simulink model "four_machine"  (R2020a)
settings: Solver=ode15s  StartTime=0.0  StopTime=20  MaxStep=1/60  RelTol=1e-3  EnableMultiTasking=on
values from neighbouring files (symbols this model uses):
  case_n = i-1    [main_simulations.m]
  d11_step = load_step_size    (= 350)    [main_simulations.m]
  d5_step = 0    [main_simulations.m]
  H = [6.5 6.5 6.175 6.175]*.75    [main_simulations.m]
  kpss = 0.2    [main_simulations.m]
  Tdelay = 0.2    [main_simulations.m]
undefined symbols (not defined in the file or in its folder): D1, d_rad, Delta, K
libraries: powerlib x49, sps_avr x4, powerlib_meascontrol x4, simulink x2, dspsigops x2
(part 2 of 2)

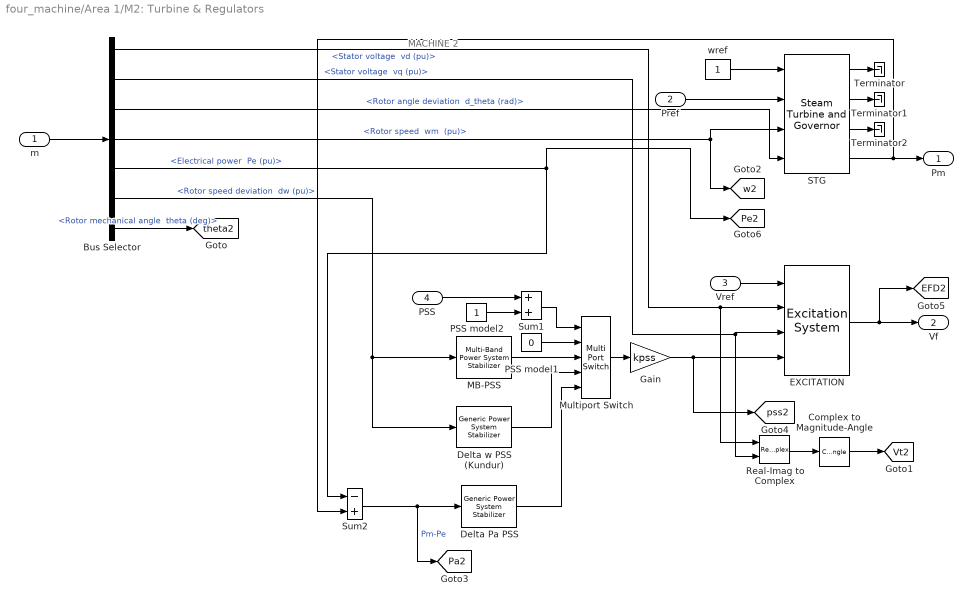
== system four_machine/Area 1/M2: Turbine & Regulators ==
  note: MACHINE 2
  m : Inport
  Pref : Inport  Port=2
  Vref : Inport  Port=3
  PSS : Inport  Port=4
  Bus Selector : BusSelector  OutputSignals="dq0 components.Stator voltage  vd (pu),dq0 components.Stator voltage  vq (pu),Mechanical.Rotor angle deviation  d_theta (rad),Mechanical.Rotor speed  wm  (pu),Mechanical.Electrical power  Pe (pu),Mechanical.Rotor speed deviation  dw (pu),Mechanical.Rotor mechanical angle  theta (deg)"
  Complex to Magnitude-Angle : ComplexToMagnitudeAngle  Output=Magnitude
  "Delta Pa PSS " : powerlib/Machines/Generic Power System Stabilizer  Tsensor=15e-3  K=2.5*1.25  Twashout=1  Tleadlag1=[60e-3 1]  Tleadlag2=[0 0]  VSlimits=[-0.15 0.15]  Vinit=0  Plot_On=off  MagdB_On=on  FreqRange=logspace(-2,2,500)
      settings: SourceProductBaseCode=PS
  "Delta w PSS (Kundur) " : powerlib/Machines/Generic Power System Stabilizer  Tsensor=15e-3  K=30  Twashout=10  Tleadlag1=[50e-3 20e-3]  Tleadlag2=[3 5.4]  VSlimits=[-0.15 0.15]  Vinit=0  Plot_On=off  MagdB_On=on  FreqRange=logspace(-2,2,500)
      settings: SourceProductBaseCode=PS
  EXCITATION : sps_avr/Excitation System  tr=20e-3  reg=[ 200, 0.001 ]  exc=[ 1, 0 ]  tgr=[ 0, 0 ]  damp=[ 0, 0 ]  sat=[ 0, 0 ]  lim=[ 0 , 12.3, 0 ]  v0=[1 2.1188]
      settings: SourceProductBaseCode=PS
  Gain : Gain  Gain=kpss
  "MB-PSS " : powerlib/Machines/Multi-Band Power System Stabilizer  OperationMode=Simplified settings  Kg=1.0  GL=[0.2 30]  GI=[1.25 40]  GH=[12.0 160]  GLd=[66 66 9.4]  TcLF=[1.667 2 0 0 0 0 2 2.4 0 0 0 0 1 1]  GId=[66 66 47.6]  TcIF=[1 1 0.25 0.3 0 0 1 1 0.3 0.36 0 0 0 0]  GHd=[66 66 233]  TcHF="[0.01 0.012 0 0 0 0  0.012 0.0144 0 0 0 0 1 1]"  LIM=[.075 .15 .15 .15]  Plot_On=off  MagdB_On=off  FreqRange=logspace(-2,2,500)
      settings: SourceProductBaseCode=PS
  Multiport Switch : MultiPortSwitch  Inputs=4  InputSameDT=on
  PSS model1 : Constant  Value=0
  PSS model2 : Constant
  Real-Imag to Complex : RealImagToComplex
  STG : powerlib/Machines/Steam Turbine and Governor  gentype=Tandem-compound (single mass)  reg1="[ 1  0.05    0 ]"  reg2="[ 0.001  0.15 ]"  reg3="[ -0.1  0.1  0  4.496 ]"  N=3600  turb1="[ 0  10   3.3   0.5   ]"  turb2="[   0   0.36    0.36   0.28   ]"  HA="[ 0.046  1.430  1.465   0.192 ]"  KA="[ 90.44  53.88  64.59   62.94  ]"  DA="[ 0.0115  0.3575  0.3663   0.0137  ]"  ini1=0.86358  ini2=[0.779243,-42.8075]
      settings: SourceProductBaseCode=PS
  Sum1 : Sum  InputSameDT=on  SaturateOnIntegerOverflow=on  OutDataTypeStr=Inherit: Same as first input
  Sum2 : Sum  Inputs=-+  InputSameDT=on  SaturateOnIntegerOverflow=on  OutDataTypeStr=Inherit: Same as first input
  Terminator : Terminator
  Terminator1 : Terminator
  Terminator2 : Terminator
  wref : Constant
  Pm : Outport  InitialOutput=0  VectorParamsAs1DForOutWhenUnconnected=off
  Vf : Outport  Port=2  InitialOutput=0  VectorParamsAs1DForOutWhenUnconnected=off
  tag scope: EFD2=global, Pa2=global, Pe2=global, Vt2=global, pss2=global, theta2=global, w2=global
  wires:
  Sum2/1 -> [Pa2], "Delta Pa PSS "/1  "Pm-Pe"
  Bus Selector/6 -> "MB-PSS "/1, "Delta w PSS (Kundur) "/1  "<Rotor speed deviation  dw (pu)>"
  Bus Selector/5 -> [Pe2], Sum2/1  "<Electrical power  Pe (pu)>"
  Bus Selector/4 -> STG/3, [w2]  "<Rotor speed  wm  (pu)>"
  PSS/1 -> Sum1/1
  Sum1/1 -> Multiport Switch/1
  PSS model2/1 -> Sum1/2
  "Delta Pa PSS "/1 -> Multiport Switch/5
  "Delta w PSS (Kundur) "/1 -> Multiport Switch/4
  "MB-PSS "/1 -> Multiport Switch/3
  PSS model1/1 -> Multiport Switch/2
  Multiport Switch/1 -> Gain/1
  Bus Selector/7 -> [theta2]  "<Rotor mechanical angle  theta (deg)>"
  Complex to Magnitude-Angle/1 -> [Vt2]
  EXCITATION/1 -> [EFD2], Vf/1
  Real-Imag to Complex/1 -> Complex to Magnitude-Angle/1
  Vref/1 -> EXCITATION/1
  Pref/1 -> STG/2
  wref/1 -> STG/1
  Bus Selector/2 -> Real-Imag to Complex/2, EXCITATION/3  "<Stator voltage  vq (pu)>"
  Bus Selector/1 -> Real-Imag to Complex/1, EXCITATION/2  "<Stator voltage  vd (pu)>"
  STG/1 -> Terminator/1
  STG/2 -> Terminator1/1
  STG/3 -> Terminator2/1
  STG/4 -> Pm/1, Sum2/2
  Bus Selector/3 -> STG/4  "<Rotor angle deviation  d_theta (rad)>"
  m/1 -> Bus Selector/1
  Gain/1 -> [pss2], EXCITATION/4

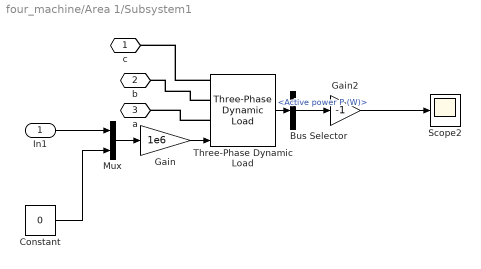
== system four_machine/Area 1/Subsystem1 ==
  In1 : Inport
  Bus Selector : BusSelector  OutputSignals=Active power P (W)
  Constant : Constant  Value=0
  Gain : Gain  Gain=1e6
  Gain2 : Gain  Gain=-1
  Mux : Mux  Inputs=2
  Scope2 : Scope
  Three-Phase Dynamic Load : powerlib/Elements/Three-Phase Dynamic Load  NominalVoltage=[ 230e3 60 ]  ActiveReactivePowers=[1e-06 1e-06]  PositiveSequence=[0.985471 32.8037]  ExternalControl=on  NpNq=[1.3 2]  TimeConstants="[0  0  0  0]"  MinimumVoltage=0.7  Tfilter=1e-4  LoadFlowParameters=[4,0,0,0,0]
      settings: SourceProductBaseCode=PS
  c : PMIOPort  Side=Left
  b : PMIOPort  Port=2  Side=Left
  a : PMIOPort  Port=3  Side=Left
  wires:
  Bus Selector/1 -> Gain2/1  "<Active power P (W)>"
  Three-Phase Dynamic Load/1 -> Bus Selector/1
  Mux/1 -> Gain/1
  Constant/1 -> Mux/2
  Gain/1 -> Three-Phase Dynamic Load/1
  In1/1 -> Mux/1
  Gain2/1 -> Scope2/1
  connections:
  Three-Phase Dynamic Load/LConn2 -- b/RConn1
  Three-Phase Dynamic Load/LConn3 -- c/RConn1
  Three-Phase Dynamic Load/LConn1 -- a/RConn1

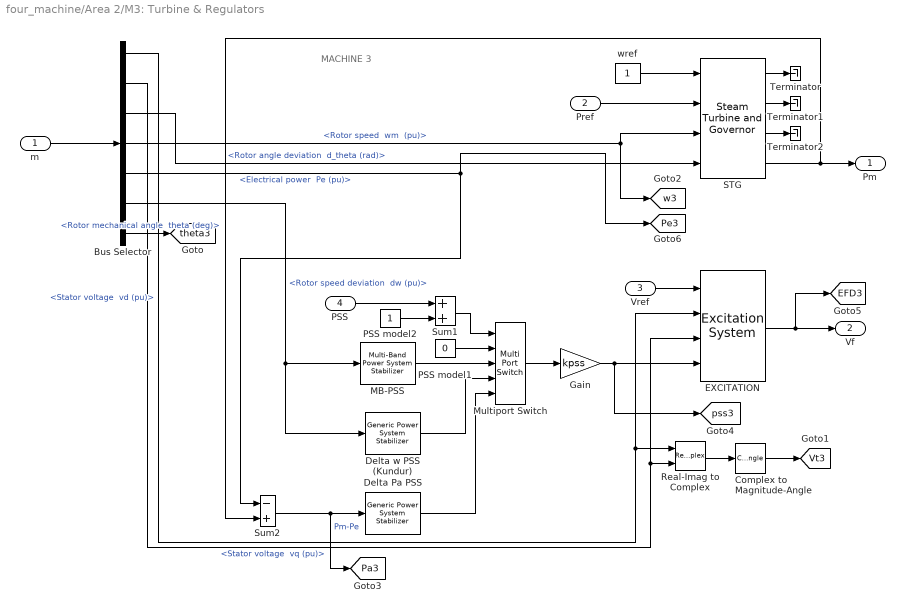
== system four_machine/Area 2/M3: Turbine & Regulators ==
  note: MACHINE 3
  m : Inport
  Pref : Inport  Port=2
  Vref : Inport  Port=3
  PSS : Inport  Port=4
  Bus Selector : BusSelector  OutputSignals="dq0 components.Stator voltage  vd (pu),dq0 components.Stator voltage  vq (pu),Mechanical.Rotor angle deviation  d_theta (rad),Mechanical.Rotor speed  wm  (pu),Mechanical.Electrical power  Pe (pu),Mechanical.Rotor speed deviation  dw (pu),Mechanical.Rotor mechanical angle  theta (deg)"
  Complex to Magnitude-Angle : ComplexToMagnitudeAngle  Output=Magnitude
  "Delta Pa PSS " : powerlib/Machines/Generic Power System Stabilizer  Tsensor=15e-3  K=2.5*1.25  Twashout=1  Tleadlag1=[60e-3 1]  Tleadlag2=[0 0]  VSlimits=[-0.15 0.15]  Vinit=0  Plot_On=off  MagdB_On=on  FreqRange=logspace(-2,2,500)
      settings: SourceProductBaseCode=PS
  "Delta w PSS (Kundur) " : powerlib/Machines/Generic Power System Stabilizer  Tsensor=15e-3  K=30  Twashout=10  Tleadlag1=[50e-3 20e-3]  Tleadlag2=[3 5.4]  VSlimits=[-0.15 0.15]  Vinit=0  Plot_On=off  MagdB_On=on  FreqRange=logspace(-2,2,500)
      settings: SourceProductBaseCode=PS
  EXCITATION : sps_avr/Excitation System  tr=20e-3  reg=[ 200, 0.001 ]  exc=[ 1, 0 ]  tgr=[ 0, 0 ]  damp=[ 0, 0 ]  sat=[ 0, 0 ]  lim=[ 0 , 12.3, 0 ]  v0=[1 1.8982]
      settings: SourceProductBaseCode=PS
  Gain : Gain  Gain=kpss
  "MB-PSS " : powerlib/Machines/Multi-Band Power System Stabilizer  OperationMode=Simplified settings  Kg=1.0  GL=[0.2 30]  GI=[1.25 40]  GH=[12.0 160]  GLd=[66 66 9.4]  TcLF=[1.667 2 0 0 0 0 2 2.4 0 0 0 0 1 1]  GId=[66 66 47.6]  TcIF=[1 1 0.25 0.3 0 0 1 1 0.3 0.36 0 0 0 0]  GHd=[66 66 233]  TcHF="[0.01 0.012 0 0 0 0  0.012 0.0144 0 0 0 0 1 1]"  LIM=[.075 .15 .15 .15]  Plot_On=off  MagdB_On=off  FreqRange=logspace(-2,2,500)
      settings: SourceProductBaseCode=PS
  Multiport Switch : MultiPortSwitch  Inputs=4  InputSameDT=on
  PSS model1 : Constant  Value=0
  PSS model2 : Constant
  Real-Imag to Complex : RealImagToComplex
  STG : powerlib/Machines/Steam Turbine and Governor  gentype=Tandem-compound (single mass)  reg1="[ 1  0.05    0 ]"  reg2="[ 0.001  0.15 ]"  reg3="[ -0.1  0.1  0  4.496 ]"  N=3600  turb1="[ 0  10   3.3   0.5   ]"  turb2="[   0   0.36    0.36   0.28   ]"  HA="[ 0.046  1.430  1.465   0.192 ]"  KA="[ 90.44  53.88  64.59   62.94  ]"  DA="[ 0.0115  0.3575  0.3663   0.0137  ]"  ini1=0.80053  ini2=[0.800505,-56.3243]
      settings: SourceProductBaseCode=PS
  Sum1 : Sum  InputSameDT=on  SaturateOnIntegerOverflow=on  OutDataTypeStr=Inherit: Same as first input
  Sum2 : Sum  Inputs=-+  InputSameDT=on  SaturateOnIntegerOverflow=on  OutDataTypeStr=Inherit: Same as first input
  Terminator : Terminator
  Terminator1 : Terminator
  Terminator2 : Terminator
  wref : Constant
  Pm : Outport  InitialOutput=0  VectorParamsAs1DForOutWhenUnconnected=off
  Vf : Outport  Port=2  InitialOutput=0  VectorParamsAs1DForOutWhenUnconnected=off
  tag scope: EFD3=global, Pa3=global, Pe3=global, Vt3=global, pss3=global, theta3=global, w3=global
  wires:
  Sum2/1 -> [Pa3], "Delta Pa PSS "/1  "Pm-Pe"
  Bus Selector/6 -> "MB-PSS "/1, "Delta w PSS (Kundur) "/1  "<Rotor speed deviation  dw (pu)>"
  Bus Selector/5 -> [Pe3], Sum2/1  "<Electrical power  Pe (pu)>"
  Bus Selector/4 -> STG/3, [w3]  "<Rotor speed  wm  (pu)>"
  PSS/1 -> Sum1/1
  Sum1/1 -> Multiport Switch/1
  PSS model2/1 -> Sum1/2
  "Delta Pa PSS "/1 -> Multiport Switch/5
  "Delta w PSS (Kundur) "/1 -> Multiport Switch/4
  "MB-PSS "/1 -> Multiport Switch/3
  PSS model1/1 -> Multiport Switch/2
  Multiport Switch/1 -> Gain/1
  Bus Selector/7 -> [theta3]  "<Rotor mechanical angle  theta (deg)>"
  Complex to Magnitude-Angle/1 -> [Vt3]
  EXCITATION/1 -> [EFD3], Vf/1
  Real-Imag to Complex/1 -> Complex to Magnitude-Angle/1
  Vref/1 -> EXCITATION/1
  Pref/1 -> STG/2
  wref/1 -> STG/1
  Bus Selector/2 -> EXCITATION/3, Real-Imag to Complex/2  "<Stator voltage  vq (pu)>"
  Bus Selector/1 -> EXCITATION/2, Real-Imag to Complex/1  "<Stator voltage  vd (pu)>"
  Bus Selector/3 -> STG/4  "<Rotor angle deviation  d_theta (rad)>"
  STG/1 -> Terminator/1
  STG/2 -> Terminator1/1
  STG/3 -> Terminator2/1
  STG/4 -> Pm/1, Sum2/2
  m/1 -> Bus Selector/1
  Gain/1 -> [pss3], EXCITATION/4

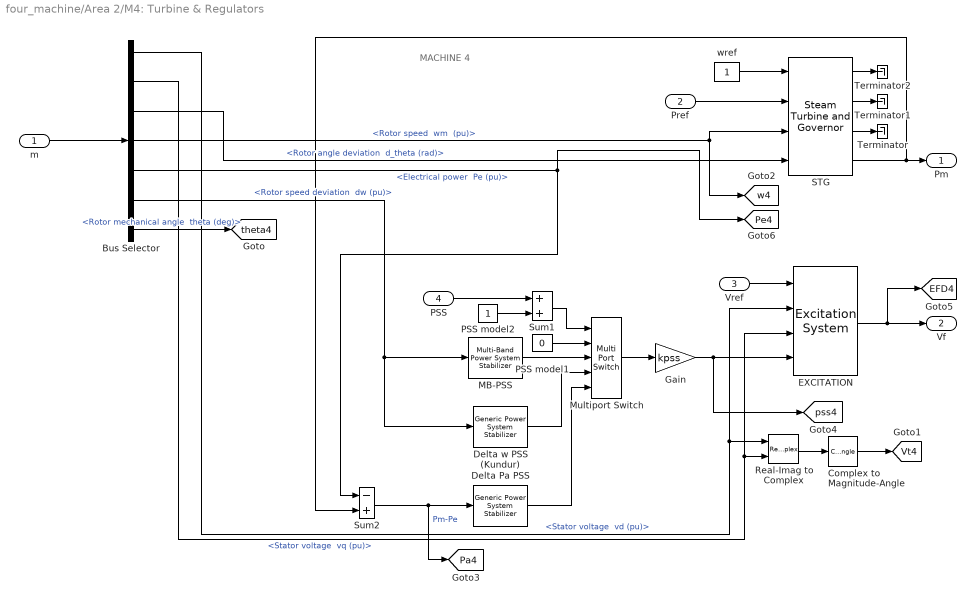
== system four_machine/Area 2/M4: Turbine & Regulators ==
  note: MACHINE 4
  m : Inport
  Pref : Inport  Port=2
  Vref : Inport  Port=3
  PSS : Inport  Port=4
  Bus Selector : BusSelector  OutputSignals="dq0 components.Stator voltage  vd (pu),dq0 components.Stator voltage  vq (pu),Mechanical.Rotor angle deviation  d_theta (rad),Mechanical.Rotor speed  wm  (pu),Mechanical.Electrical power  Pe (pu),Mechanical.Rotor speed deviation  dw (pu),Mechanical.Rotor mechanical angle  theta (deg)"
  Complex to Magnitude-Angle : ComplexToMagnitudeAngle  Output=Magnitude
  "Delta Pa PSS " : powerlib/Machines/Generic Power System Stabilizer  Tsensor=15e-3  K=2.5*1.25  Twashout=1  Tleadlag1=[60e-3 1]  Tleadlag2=[0 0]  VSlimits=[-0.15 0.15]  Vinit=0  Plot_On=off  MagdB_On=on  FreqRange=logspace(-2,2,500)
      settings: SourceProductBaseCode=PS
  "Delta w PSS (Kundur) " : powerlib/Machines/Generic Power System Stabilizer  Tsensor=15e-3  K=30  Twashout=10  Tleadlag1=[50e-3 20e-3]  Tleadlag2=[3 5.4]  VSlimits=[-0.15 0.15]  Vinit=0  Plot_On=off  MagdB_On=on  FreqRange=logspace(-2,2,500)
      settings: SourceProductBaseCode=PS
  EXCITATION : sps_avr/Excitation System  tr=20e-3  reg=[ 200, 0.001 ]  exc=[ 1, 0 ]  tgr=[ 0, 0 ]  damp=[ 0, 0 ]  sat=[ 0, 0 ]  lim=[ 0 , 12.3, 0 ]  v0=[1 1.9423]
      settings: SourceProductBaseCode=PS
  Gain : Gain  Gain=kpss
  "MB-PSS " : powerlib/Machines/Multi-Band Power System Stabilizer  OperationMode=Simplified settings  Kg=1.0  GL=[0.2 30]  GI=[1.25 40]  GH=[12.0 160]  GLd=[66 66 9.4]  TcLF=[1.667 2 0 0 0 0 2 2.4 0 0 0 0 1 1]  GId=[66 66 47.6]  TcIF=[1 1 0.25 0.3 0 0 1 1 0.3 0.36 0 0 0 0]  GHd=[66 66 233]  TcHF="[0.01 0.012 0 0 0 0  0.012 0.0144 0 0 0 0 1 1]"  LIM=[.075 .15 .15 .15]  Plot_On=off  MagdB_On=off  FreqRange=logspace(-2,2,500)
      settings: SourceProductBaseCode=PS
  Multiport Switch : MultiPortSwitch  Inputs=4  InputSameDT=on
  PSS model1 : Constant  Value=0
  PSS model2 : Constant
  Real-Imag to Complex : RealImagToComplex
  STG : powerlib/Machines/Steam Turbine and Governor  gentype=Tandem-compound (single mass)  reg1="[ 1  0.05    0 ]"  reg2="[ 0.001  0.15 ]"  reg3="[ -0.1  0.1  0  4.496 ]"  N=3600  turb1="[ 0  10   3.3   0.5   ]"  turb2="[   0   0.36    0.36   0.28   ]"  HA="[ 0.046  1.430  1.465   0.192 ]"  KA="[ 90.44  53.88  64.59   62.94  ]"  DA="[ 0.0115  0.3575  0.3663   0.0137  ]"  ini1=0.77938  ini2=[0.779311,-67.7513]
      settings: SourceProductBaseCode=PS
  Sum1 : Sum  InputSameDT=on  SaturateOnIntegerOverflow=on  OutDataTypeStr=Inherit: Same as first input
  Sum2 : Sum  Inputs=-+  InputSameDT=on  SaturateOnIntegerOverflow=on  OutDataTypeStr=Inherit: Same as first input
  Terminator : Terminator
  Terminator1 : Terminator
  Terminator2 : Terminator
  wref : Constant
  Pm : Outport  InitialOutput=0  VectorParamsAs1DForOutWhenUnconnected=off
  Vf : Outport  Port=2  InitialOutput=0  VectorParamsAs1DForOutWhenUnconnected=off
  tag scope: EFD4=global, Pa4=global, Pe4=global, Vt4=global, pss4=global, theta4=global, w4=global
  wires:
  Bus Selector/1 -> EXCITATION/2, Real-Imag to Complex/1  "<Stator voltage  vd (pu)>"
  Bus Selector/2 -> EXCITATION/3, Real-Imag to Complex/2  "<Stator voltage  vq (pu)>"
  STG/4 -> Pm/1, Sum2/2
  wref/1 -> STG/1
  Pref/1 -> STG/2
  Vref/1 -> EXCITATION/1
  STG/3 -> Terminator/1
  Real-Imag to Complex/1 -> Complex to Magnitude-Angle/1
  EXCITATION/1 -> Vf/1, [EFD4]
  Complex to Magnitude-Angle/1 -> [Vt4]
  Bus Selector/7 -> [theta4]  "<Rotor mechanical angle  theta (deg)>"
  Multiport Switch/1 -> Gain/1
  PSS model1/1 -> Multiport Switch/2
  "MB-PSS "/1 -> Multiport Switch/3
  "Delta w PSS (Kundur) "/1 -> Multiport Switch/4
  "Delta Pa PSS "/1 -> Multiport Switch/5
  PSS model2/1 -> Sum1/2
  Sum1/1 -> Multiport Switch/1
  PSS/1 -> Sum1/1
  Bus Selector/4 -> STG/3, [w4]  "<Rotor speed  wm  (pu)>"
  Bus Selector/5 -> [Pe4], Sum2/1  "<Electrical power  Pe (pu)>"
  Bus Selector/6 -> "MB-PSS "/1, "Delta w PSS (Kundur) "/1  "<Rotor speed deviation  dw (pu)>"
  Sum2/1 -> [Pa4], "Delta Pa PSS "/1  "Pm-Pe"
  STG/2 -> Terminator1/1
  STG/1 -> Terminator2/1
  Bus Selector/3 -> STG/4  "<Rotor angle deviation  d_theta (rad)>"
  m/1 -> Bus Selector/1
  Gain/1 -> EXCITATION/4, [pss4]

== system four_machine/Area 2/Subsystem1 ==
  In1 : Inport
  Bus Selector : BusSelector  OutputSignals=Active power P (W)
  Constant : Constant  Value=0
  Gain : Gain  Gain=1e6
  Gain2 : Gain  Gain=-1
  Mux : Mux  Inputs=2
  Scope2 : Scope
  Three-Phase Dynamic Load : powerlib/Elements/Three-Phase Dynamic Load  NominalVoltage=[ 230e3 60 ]  ActiveReactivePowers=[1e-06 1e-06]  PositiveSequence=[0.98771 -4.64632]  ExternalControl=on  NpNq=[1.3 2]  TimeConstants="[0  0  0  0]"  MinimumVoltage=0.7  Tfilter=1e-4  LoadFlowParameters=[4,0,0,0,0]
      settings: SourceProductBaseCode=PS
  c : PMIOPort  Side=Left
  b : PMIOPort  Port=2  Side=Left
  a : PMIOPort  Port=3  Side=Left
  wires:
  Bus Selector/1 -> Gain2/1  "<Active power P (W)>"
  Three-Phase Dynamic Load/1 -> Bus Selector/1
  Mux/1 -> Gain/1
  Constant/1 -> Mux/2
  Gain/1 -> Three-Phase Dynamic Load/1
  In1/1 -> Mux/1
  Gain2/1 -> Scope2/1
  connections:
  Three-Phase Dynamic Load/LConn2 -- b/RConn1
  Three-Phase Dynamic Load/LConn3 -- c/RConn1
  Three-Phase Dynamic Load/LConn1 -- a/RConn1

== system four_machine/Subsystem3/Subsystem ==
  u : Inport
  Enable : EnablePort
  y : Outport  VectorParamsAs1DForOutWhenUnconnected=off
  wires:
  u/1 -> y/1

== system four_machine/Subsystem4/Subsystem ==
  u : Inport
  Enable : EnablePort
  y : Outport  VectorParamsAs1DForOutWhenUnconnected=off
  wires:
  u/1 -> y/1

== system four_machine/Subsystem5/Subsystem ==
  u : Inport
  Enable : EnablePort
  y : Outport  VectorParamsAs1DForOutWhenUnconnected=off
  wires:
  u/1 -> y/1

== system four_machine/System Data/Subsystem3 ==
  input : Inport
  Step2 : Step  Time=1e-9  Before=1  After=0  SampleTime=0  ZeroCross=off
  Subsystem : Subsystem  AncestorBlock="Nordic32_Lib/PSS  Nordic32/Subsystem"
  Subtract : Sum  Inputs=+-
  output : Outport  VectorParamsAs1DForOutWhenUnconnected=off
  wires:
  Step2/1 -> Subsystem/Enable
  Subsystem/1(y) -> Subtract/2  "Pe0"
  input/1 -> Subtract/1, Subsystem/1(u)
  Subtract/1 -> output/1

== system four_machine/System Data/Subsystem3/Subsystem ==
  u : Inport
  Enable : EnablePort
  y : Outport  VectorParamsAs1DForOutWhenUnconnected=off
  wires:
  u/1 -> y/1
